simulink model "Ctrl_Kjerstad_DP_1"  (R2014a)
settings: Solver=ode4  StartTime=0.0  StopTime=inf  FixedStep=0.01  RelTol=1e-3
(part 2 of 2)

== matlab function Ctrl_Kjerstad_DP_1/Control law/Tau PD-control/Integral  gain/diag3x3 ==
  data: u input; y output
function y = fcn(u)


y = diag([u(1) u(2) u(3)]);

== matlab function Ctrl_Kjerstad_DP_1/Control law/Tau PD-control/Proportional gain/diag3x3 ==
  data: u input; y output
function y = fcn(u)


y = diag([u(1) u(2) u(3)]);

== matlab function Ctrl_Kjerstad_DP_1/Control law/Tau PD-control/Derivative gain/diag3x3 ==
  data: u input; y output
function y = fcn(u)


y = diag([u(1) u(2) u(3)]);

== matlab function Ctrl_Kjerstad_DP_1/Thruster allocation/Thrust allocation ==
  data: tau_x input; u_BT output; tau_y input; tau_psi input; l_BT input; l_VSP input; u_VSP output; alpha_VSP output
function [u_BT,u_VSP,alpha_VSP] = fcn(tau_x,tau_y,tau_psi,l_BT,l_VSP)

tau_trans = abs(tau_x) + abs(tau_y);

u_VSP_trans     = tau_trans;
alpha_VSP_trans = atan2(tau_y,tau_x);
u_BT_trans      = tau_trans*sin(alpha_VSP_trans)*l_VSP/l_BT;

u_VSP_rot     = abs(tau_psi)      /l_VSP;
alpha_VSP_rot = sign(-tau_psi)*pi/2;
u_BT_rot      = tau_psi           /l_BT;

u_VSP     = u_VSP_trans + u_VSP_rot;
alpha_VSP = alpha_VSP_trans + alpha_VSP_rot;
u_BT      = u_BT_trans + u_BT_rot;
